simulink model "flow_sns"  (R2022a)
settings: Solver=FixedStepAuto  StartTime=0.0  StopTime=15  RelTol=1e-3  EnableMultiTasking=on
libraries: simulink x7, hdlsllib x4, mbedblockslib x3
settings Model: SimulationMode=external  ExtModeTrigDuration=10  Creator=FUGAZI  LastModifiedBy=smith
settings OptimizationCC: EnhancedBackFolding=on  PassReuseOutputArgsAs=Individual arguments  ZeroExternalMemoryAtStartup=off  ZeroInternalMemoryAtStartup=off  MaxStackSize=64  OptimizeBlockOrder=speed  DifferentSizesBufferReuse=on  OptimizationCustomize=off  EfficientTunableParamExpr=on
settings DebuggingCC: ParameterTunabilityLossMsg=error
settings HardwareCC: ProdBitPerPointer=32  ProdBitPerSizeT=32  ProdBitPerPtrDiffT=32  ProdLargestAtomicInteger=Long  ProdLargestAtomicFloat=Double  ProdWordSize=32  ProdLongLongMode=on  ProdHWDeviceType=ARM Compatible->ARM Cortex
settings SFSimCC: MATLABDynamicMemAlloc=off
settings RTWCC: SystemTargetFile=ert.tlc  HardwareBoard=STM32 Nucleo L476RG  TemplateMakefile=ert_default_tmf  Toolchain=GNU Tools for ARM Embedded Processors
settings CodeAppCC: ForceParamTrailComments=on  IgnoreCustomStorageClasses=off  OperatorAnnotations=on  SimulinkDataObjDesc=on  SFDataObjDesc=on  InsertBlockDesc=on
settings ERTTargetCC: SupportContinuousTime=on  ExtMode=on  ExtModeTransport=3  ExtModeStaticAlloc=on  ExtModeStaticAllocSize=2000  ExtModeMexFile=ext_xcp  ExtModeMexArgs=1 4 115200  ExtModeIntrfLevel=Level2 - Open

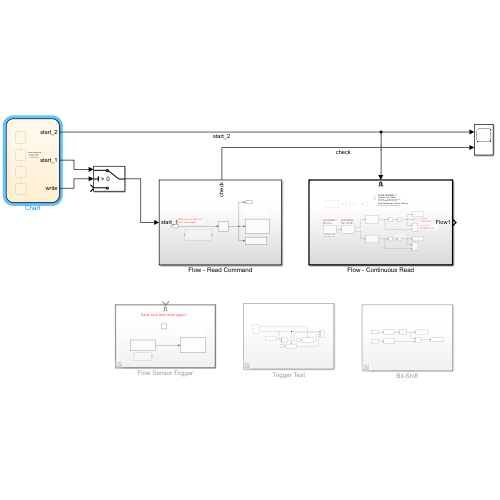
[thumbnail: Simulink's stored preview of the top-level diagram]
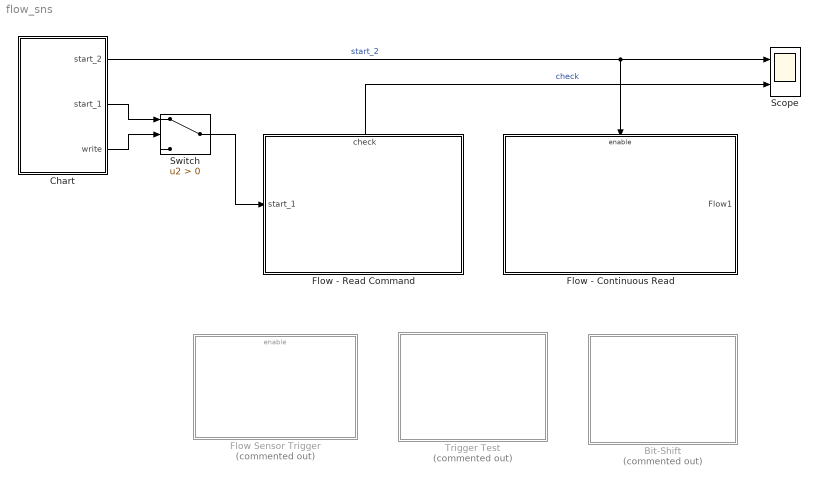
== system flow_sns ==
  Bit-Shift : Subsystem  Commented=on
  Chart : Stateflow chart  TreatAsAtomicUnit=on
      settings: PortSchema="{\"entries\":[{\"content\":{\"sides\":[{\"content\":{\"connectorIds\":[]},\"type\":\"ConnectorPlacement.EquallySpacedRectSide\",\"uuid\":\"751ec28f-069a-417f-8b9c-26d70f125eaf\"},{\"content\":{\"connectorIds\":[\"Out2\",\"Out1\",\"Out3\"],\"side\":\"RIGHT\"},\"type\":\"ConnectorPlacement.EquallySpacedRectSide\",\"uuid\":\"74ecb3a5-1f56-41c3-8a4c-212d8a69cc27\"},{\"content\":{\"connectorIds\":[],\"side\":\"TOP\"},\"type\":\"ConnectorPlacement.EquallySpacedRectSide\",\"uuid\":\"ea9723c7-ae57-446b-9b85-bce3bac5bf5f\"}]},\"type\":\"ConnectorPlacement.EquallySpacedConnector\",\"uuid\":\"1a0f9f5c-2546-4b71-a73d-7ce3ff689e76\"}],\"packageUris\":[\"http://schema.mathworks.com/mf0/Connector/R2020b\"],\"version\":\"1.0\"}"
  Flow - Continuous Read : Subsystem
  Flow - Read Command : Subsystem
      settings: PortSchema="{\"entries\":[{\"content\":{\"sides\":[{\"content\":{\"connectorIds\":[\"In1\"]},\"type\":\"ConnectorPlacement.EquallySpacedRectSide\",\"uuid\":\"93933be5-5d1d-4e29-9d84-8c5fcd33ad64\"},{\"content\":{\"connectorIds\":[],\"side\":\"RIGHT\"},\"type\":\"ConnectorPlacement.EquallySpacedRectSide\",\"uuid\":\"5f3334d1-31af-43f4-9ed8-c3b8fb739727\"},{\"content\":{\"connectorIds\":[\"Out1\"],\"side\":\"TOP\"},\"type\":\"ConnectorPlacement.EquallySpacedRectSide\",\"uuid\":\"aa0caa1c-490f-4eb3-a1f0-284b936a223e\"}]},\"type\":\"ConnectorPlacement.EquallySpacedConnector\",\"uuid\":\"c416ffdc-2385-461c-9877-3be2c663fd49\"}],\"packageUris\":[\"http://schema.mathworks.com/mf0/Connector/R2020b\"],\"version\":\"1.0\"}"
  Flow Sensor Trigger : Subsystem  Commented=on
  Scope : Scope  NumInputPorts=2
  Switch : Switch  Criteria=u2 > Threshold  SaturateOnIntegerOverflow=off  InputSameDT=off
  Trigger Test : Subsystem  Commented=on
  wires:
  Chart/1(start_1) -> Switch/1
  Chart/2(start_2) -> Flow - Continuous Read/Enable, Scope/1  "start_2"
  Switch/1 -> Flow - Read Command/1(start_1)
  Chart/3(write) -> Switch/2
  Flow - Read Command/1(check) -> Scope/2  "check"

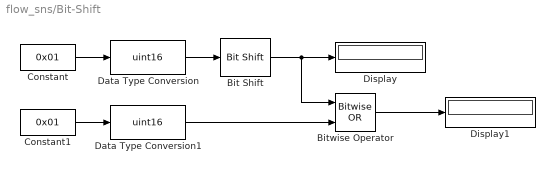
== system flow_sns/Bit-Shift ==
  Bit Shift : hdlsllib/Logic and Bit Operations/Bit Shift  mode=Shift Left Logical  N=8
  Bitwise Operator : simulink/Logic and Bit Operations/Bitwise Operator  logicop=OR  UseBitMask=off  NumInputPorts=2  BitMask=bin2dec('11011001')  BitMaskRealWorld=Stored Integer
  Constant : Constant  Value=0x01  SampleTime=0.1
  Constant1 : Constant  Value=0x01  SampleTime=0.1
  Data Type Conversion : DataTypeConversion  OutDataTypeStr=uint16  SaturateOnIntegerOverflow=off  RndMeth=Floor
  Data Type Conversion1 : DataTypeConversion  OutDataTypeStr=uint16  SaturateOnIntegerOverflow=off  RndMeth=Floor
  Display : Display
      settings: Format=hex (Stored Integer)
  Display1 : Display
      settings: Format=hex (Stored Integer)
  wires:
  Constant/1 -> Data Type Conversion/1
  Bit Shift/1 -> Bitwise Operator/1, Display/1
  Data Type Conversion/1 -> Bit Shift/1
  Constant1/1 -> Data Type Conversion1/1
  Bitwise Operator/1 -> Display1/1
  Data Type Conversion1/1 -> Bitwise Operator/2

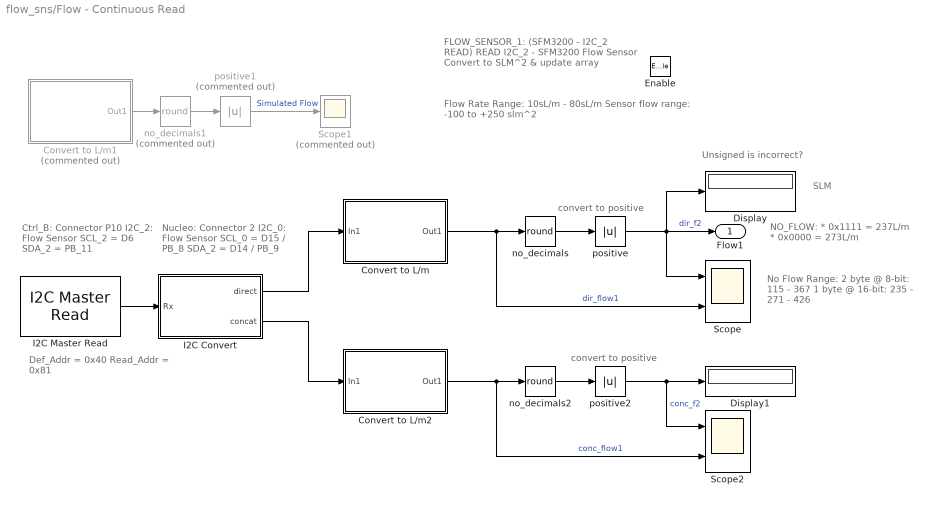
== system flow_sns/Flow - Continuous Read ==
  note: Unsigned is incorrect?
  note: NO_FLOW:
      | * 0x1111 = 237L/m
      | * 0x0000 = 273L/m
  note: Def_Addr = 0x40
      | Read_Addr = 0x81
  note: Ctrl_B: Connector P10
      | I2C_2: Flow Sensor
      | SCL_2 = D6
      | SDA_2 = PB_11
  note: FLOW_SENSOR_1:
      | (SFM3200 - I2C_2 READ)
      | READ I2C_2 - SFM3200 Flow Sensor
      | Convert to SLM^2 & update array
  note: SLM
  note: convert to positive
  note: Flow Rate Range: 10sL/m - 80sL/m
      | Sensor flow range: -100 to +250 slm^2
  note: Nucleo: Connector 2
      | I2C_0: Flow Sensor
      | SCL_0 = D15 / PB_8
      | SDA_2 = D14 / PB_9
  note: No Flow Range:
      | 2 byte @ 8-bit: 115 - 367
      | 1 byte @ 16-bit: 235 - 271 - 426
  note: convert to positive
  Enable : EnablePort
  Convert to L/m : Subsystem
  Convert to L/m1 : Subsystem  Commented=on
  Convert to L/m2 : Subsystem
  Display : Display
  Display1 : Display
  I2C Convert : Subsystem
  I2C Master Read : mbedblockslib/I2C Master Read  I2CModule=0  Mode=Master  SlaveAddress=hex2dec('81')  SlaveByteOrder=BigEndian  Direction=Receiver  RegisterAddressMode=off  RegisterAddress=uint8(0)  SlaveDataType=uint8  DataLength=3  NoAck=off  RepeatedStart=off  OutputStatus=off  SampleTime=0.1
      settings: SourceProductBaseCode=MICROBIT,NUCLEO,STMICRODIS
  Scope : Scope  NumInputPorts=2
  Scope1 : Scope  Commented=on
  Scope2 : Scope  NumInputPorts=2
  no_decimals : Rounding  Operator=round
  no_decimals1 : Rounding  Commented=on  Operator=round
  no_decimals2 : Rounding  Operator=round
  positive : Abs  SaturateOnIntegerOverflow=off
  positive1 : Abs  Commented=on  SaturateOnIntegerOverflow=off
  positive2 : Abs  SaturateOnIntegerOverflow=off
  Flow1 : Outport
  wires:
  no_decimals/1 -> positive/1
  positive/1 -> Display/1, Flow1/1, Scope/1  "dir_f2"
  I2C Master Read/1 -> I2C Convert/1(Rx)
  I2C Convert/1(direct) -> Convert to L/m/1(In1)
  Convert to L/m/1(Out1) -> Scope/2, no_decimals/1  "dir_flow1"
  no_decimals1/1 -> positive1/1
  Convert to L/m1/1(Out1) -> no_decimals1/1
  positive1/1 -> Scope1/1  "Simulated Flow"
  Convert to L/m2/1(Out1) -> Scope2/2, no_decimals2/1  "conc_flow1"
  I2C Convert/2(concat) -> Convert to L/m2/1(In1)
  no_decimals2/1 -> positive2/1
  positive2/1 -> Display1/1, Scope2/1  "conc_f2"

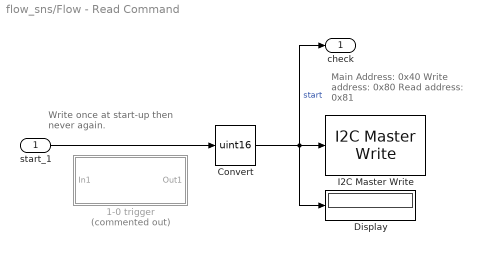
== system flow_sns/Flow - Read Command ==
  note: Main Address: 0x40
      | Write address: 0x80
      | Read address: 0x81
  note: Write once at start-up
      | then never again.
  start_1 : Inport
  1-0 trigger : Subsystem  Commented=on
  Convert : DataTypeConversion  OutDataTypeStr=uint16  RndMeth=Nearest  SaturateOnIntegerOverflow=off
  Display : Display
      settings: Format=hex (Stored Integer)
  I2C Master Write : mbedblockslib/I2C Master Write  I2CModule=0  Mode=Master  SlaveAddress=hex2dec('80')  SlaveByteOrder=BigEndian  Direction=Transmitter  RegisterAddressMode=off  RegisterAddress=uint8(1)  SlaveDataType=uint8  DataLength=2  NoAck=off  RepeatedStart=off  OutputStatus=off
      settings: SourceProductBaseCode=MICROBIT,NUCLEO,STMICRODIS
  check : Outport
  wires:
  start_1/1 -> Convert/1
  Convert/1 -> check/1, Display/1, I2C Master Write/1  "start"

== system flow_sns/Flow Sensor Trigger ==
  note: Send once then never again?
  note: Start continuous measurement
  note: Main Address: 0x40
      | Write address: 0x80
      | Read address: 0x81
  Enable : EnablePort
  Constant : Constant  Commented=on  Value=0x1000  SampleTime=-1
  Constant1 : Constant  Value=hex2dec('1000')  OutDataTypeStr=uint16
  I2C Master Write : mbedblockslib/I2C Master Write  I2CModule=0  Mode=Master  SlaveAddress=hex2dec('80')  SlaveByteOrder=BigEndian  Direction=Transmitter  RegisterAddressMode=off  RegisterAddress=uint8(1)  SlaveDataType=uint8  DataLength=2  NoAck=on  RepeatedStart=off  OutputStatus=off
      settings: SourceProductBaseCode=MICROBIT,NUCLEO,STMICRODIS
  wires:
  Constant1/1 -> I2C Master Write/1

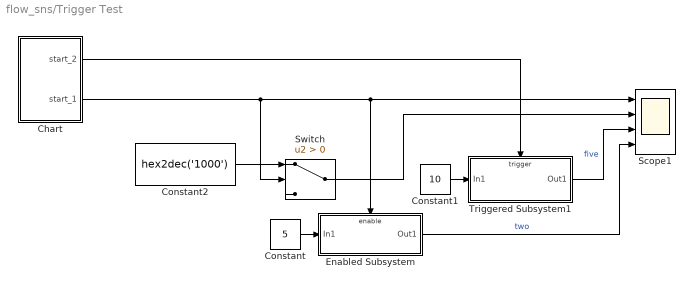
== system flow_sns/Trigger Test ==
  Chart : Stateflow chart  TreatAsAtomicUnit=on
      settings: PortSchema="{\"entries\":[{\"content\":{\"sides\":[{\"content\":{\"connectorIds\":[]},\"type\":\"ConnectorPlacement.EquallySpacedRectSide\",\"uuid\":\"751ec28f-069a-417f-8b9c-26d70f125eaf\"},{\"content\":{\"connectorIds\":[\"Out2\",\"Out1\"],\"side\":\"RIGHT\"},\"type\":\"ConnectorPlacement.EquallySpacedRectSide\",\"uuid\":\"74ecb3a5-1f56-41c3-8a4c-212d8a69cc27\"},{\"content\":{\"connectorIds\":[],\"side\":\"TOP\"},\"type\":\"ConnectorPlacement.EquallySpacedRectSide\",\"uuid\":\"ea9723c7-ae57-446b-9b85-bce3bac5bf5f\"}]},\"type\":\"ConnectorPlacement.EquallySpacedConnector\",\"uuid\":\"1a0f9f5c-2546-4b71-a73d-7ce3ff689e76\"}],\"packageUris\":[\"http://schema.mathworks.com/mf0/Connector/R2020b\"],\"version\":\"1.0\"}"
  Constant : Constant  Value=5
  Constant1 : Constant  Value=10
  Constant2 : Constant  Value=hex2dec('1000')  OutDataTypeStr=uint16
  Enabled Subsystem : Subsystem  TreatAsAtomicUnit=on
  Scope1 : Scope  NumInputPorts=4
  Switch : Switch  Criteria=u2 > Threshold  SaturateOnIntegerOverflow=off  InputSameDT=off
  Triggered Subsystem1 : Subsystem  TreatAsAtomicUnit=on
  wires:
  Constant/1 -> Enabled Subsystem/1(In1)
  Chart/2(start_2) -> Triggered Subsystem1/Trigger
  Constant1/1 -> Triggered Subsystem1/1(In1)
  Constant2/1 -> Switch/1
  Chart/1(start_1) -> Switch/2, Scope1/1, Enabled Subsystem/Enable
  Switch/1 -> Scope1/2
  Triggered Subsystem1/1(Out1) -> Scope1/3  "five"
  Enabled Subsystem/1(Out1) -> Scope1/4  "two"

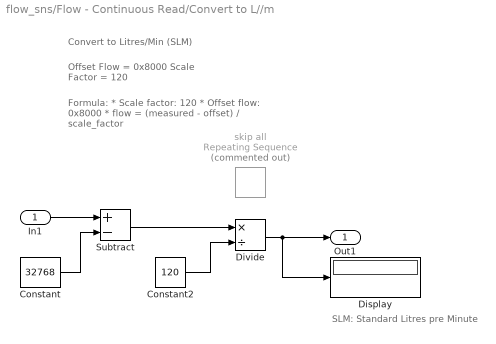
== system flow_sns/Flow - Continuous Read/Convert to L//m ==
  note: SLM: Standard Litres pre Minute
  note: Convert to Litres/Min (SLM)
  note: Offset Flow = 0x8000
      | Scale Factor = 120
  note: Formula:
      | * Scale factor: 120
      | * Offset flow: 0x8000
      | * flow = (measured - offset) / scale_factor
  In1 : Inport
  Constant : Constant  Value=32768
  Constant2 : Constant  Value=120
  Display : Display
  Divide : Product  Inputs=*/
  Subtract : Sum  Inputs=+-
  skip all : simulink/Sources/Repeating Sequence  Commented=on  rep_seq_t=[0 1.3 1.31 2.5 2.51]  rep_seq_y=[30 30 150 150 30]
  Out1 : Outport
  wires:
  Divide/1 -> Display/1, Out1/1
  Subtract/1 -> Divide/1
  Constant2/1 -> Divide/2
  Constant/1 -> Subtract/2
  In1/1 -> Subtract/1

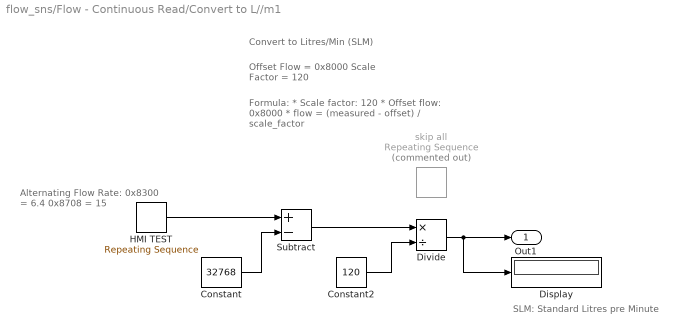
== system flow_sns/Flow - Continuous Read/Convert to L//m1 ==
  note: Formula:
      | * Scale factor: 120
      | * Offset flow: 0x8000
      | * flow = (measured - offset) / scale_factor
  note: Offset Flow = 0x8000
      | Scale Factor = 120
  note: Convert to Litres/Min (SLM)
  note: SLM: Standard Litres pre Minute
  note: Alternating Flow Rate:
      | 0x8300 = 6.4
      | 0x8708 = 15
  Constant : Constant  Value=32768
  Constant2 : Constant  Value=120
  Display : Display
  Divide : Product  Inputs=*/
  HMI TEST : simulink/Sources/Repeating Sequence  rep_seq_t=[0 2 2.05 4]  rep_seq_y=[0x8300 0x8300 0x8708 0x8708]
  Subtract : Sum  Inputs=+-
  skip all : simulink/Sources/Repeating Sequence  Commented=on  rep_seq_t=[0 1.3 1.31 2.5 2.51]  rep_seq_y=[30 30 150 150 30]
  Out1 : Outport
  wires:
  HMI TEST/1 -> Subtract/1
  Constant/1 -> Subtract/2
  Constant2/1 -> Divide/2
  Subtract/1 -> Divide/1
  Divide/1 -> Out1/1, Display/1

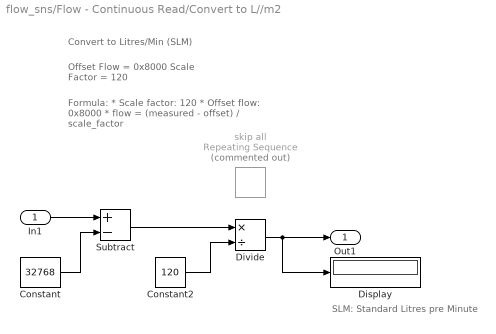
== system flow_sns/Flow - Continuous Read/Convert to L//m2 ==
  note: Formula:
      | * Scale factor: 120
      | * Offset flow: 0x8000
      | * flow = (measured - offset) / scale_factor
  note: Offset Flow = 0x8000
      | Scale Factor = 120
  note: Convert to Litres/Min (SLM)
  note: SLM: Standard Litres pre Minute
  In1 : Inport
  Constant : Constant  Value=32768
  Constant2 : Constant  Value=120
  Display : Display
  Divide : Product  Inputs=*/
  Subtract : Sum  Inputs=+-
  skip all : simulink/Sources/Repeating Sequence  Commented=on  rep_seq_t=[0 1.3 1.31 2.5 2.51]  rep_seq_y=[30 30 150 150 30]
  Out1 : Outport
  wires:
  In1/1 -> Subtract/1
  Constant/1 -> Subtract/2
  Constant2/1 -> Divide/2
  Subtract/1 -> Divide/1
  Divide/1 -> Out1/1, Display/1

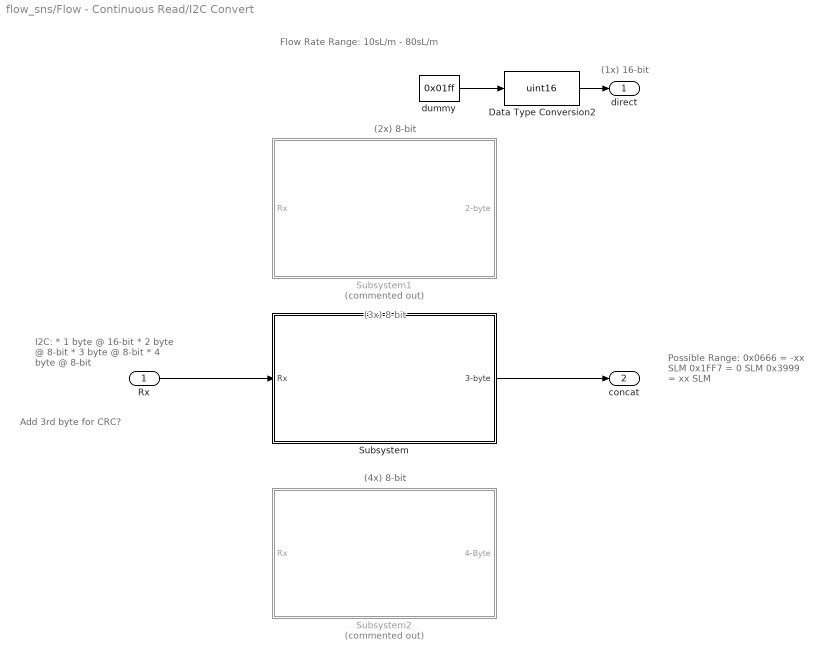
== system flow_sns/Flow - Continuous Read/I2C Convert ==
  note: (2x) 8-bit
  note: Possible Range:
      | 0x0666 = -xx SLM
      | 0x1FF7 = 0 SLM
      | 0x3999 = xx SLM
  note: Flow Rate Range: 10sL/m - 80sL/m
  note: I2C:
      | * 1 byte @ 16-bit
      | * 2 byte @ 8-bit
      | * 3 byte @ 8-bit
      | * 4 byte @ 8-bit
  note: (1x) 16-bit
  note: Add 3rd byte for CRC?
  note: (3x) 8-bit
  note: (4x) 8-bit
  Rx : Inport
  Data Type Conversion2 : DataTypeConversion  OutDataTypeStr=uint16  SaturateOnIntegerOverflow=off  RndMeth=Floor
  Subsystem : Subsystem
  Subsystem1 : Subsystem  Commented=on
  Subsystem2 : Subsystem  Commented=on
  dummy : Constant  Value=0x01ff
  direct : Outport
  concat : Outport  Port=2
  wires:
  Data Type Conversion2/1 -> direct/1
  dummy/1 -> Data Type Conversion2/1
  Rx/1 -> Subsystem/1(Rx)
  Subsystem/1(3-byte) -> concat/1

== system flow_sns/Flow - Read Command/1-0 trigger ==
  In1 : Inport
  Trigger Write : Switch  Criteria=u2 > Threshold  SaturateOnIntegerOverflow=off  InputSameDT=off
  dec(4096) : Constant  Value=hex2dec('1000')  OutDataTypeStr=uint16  SampleTime=0.1
  Out1 : Outport
  wires:
  dec(4096)/1 -> Trigger Write/1
  In1/1 -> Trigger Write/2
  Trigger Write/1 -> Out1/1

== system flow_sns/Trigger Test/Enabled Subsystem ==
  In1 : Inport
  Enable : EnablePort  StatesWhenEnabling=reset
  Out1 : Outport
  wires:
  In1/1 -> Out1/1

== system flow_sns/Trigger Test/Triggered Subsystem1 ==
  In1 : Inport
  Trigger : TriggerPort  VariantControl=(inherit)
  Constant : Constant  Value=5
  Out1 : Outport
  wires:
  In1/1 -> Out1/1

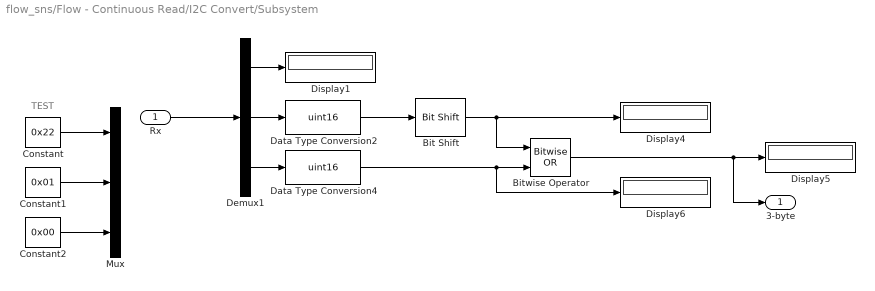
== system flow_sns/Flow - Continuous Read/I2C Convert/Subsystem ==
  note: TEST
  Rx : Inport
  Bit Shift : hdlsllib/Logic and Bit Operations/Bit Shift  mode=Shift Left Logical  N=8
  Bitwise Operator : simulink/Logic and Bit Operations/Bitwise Operator  logicop=OR  UseBitMask=off  NumInputPorts=2  BitMask=bin2dec('11011001')  BitMaskRealWorld=Stored Integer
  Constant : Constant  Value=0x22
  Constant1 : Constant  Value=0x01
  Constant2 : Constant  Value=0x00
  Data Type Conversion2 : DataTypeConversion  OutDataTypeStr=uint16  SaturateOnIntegerOverflow=off  RndMeth=Floor
  Data Type Conversion4 : DataTypeConversion  OutDataTypeStr=uint16  SaturateOnIntegerOverflow=off  RndMeth=Floor
  Demux1 : Demux  Outputs=3
  Display{1,4..6} (4 alike) : Display
      settings: Format=hex (Stored Integer)
  Mux : Mux  Inputs=3
  3-byte : Outport
  wires:
  Constant1/1 -> Mux/2
  Bit Shift/1 -> Bitwise Operator/1, Display4/1
  Demux1/3 -> Data Type Conversion4/1
  Data Type Conversion4/1 -> Display6/1, Bitwise Operator/2
  Bitwise Operator/1 -> 3-byte/1, Display5/1
  Data Type Conversion2/1 -> Bit Shift/1
  Demux1/2 -> Data Type Conversion2/1
  Demux1/1 -> Display1/1
  Constant2/1 -> Mux/3
  Constant/1 -> Mux/1
  Rx/1 -> Demux1/1

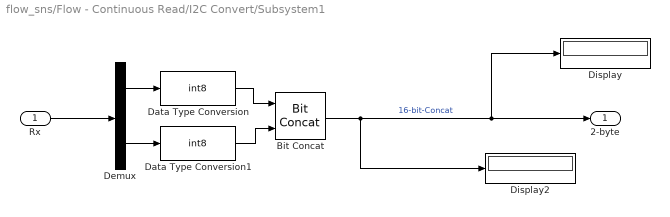
== system flow_sns/Flow - Continuous Read/I2C Convert/Subsystem1 ==
  Rx : Inport
  Bit Concat : hdlsllib/Logic and Bit Operations/Bit Concat  numInputs=2
  Data Type Conversion : DataTypeConversion  OutDataTypeStr=int8  SaturateOnIntegerOverflow=off  RndMeth=Floor
  Data Type Conversion1 : DataTypeConversion  OutDataTypeStr=int8  SaturateOnIntegerOverflow=off  RndMeth=Floor
  Demux : Demux  Outputs=2
  Display : Display
      settings: Format=hex (Stored Integer)
  Display2 : Display
      settings: Format=hex (Stored Integer)
  2-byte : Outport
  wires:
  Demux/2 -> Data Type Conversion1/1
  Bit Concat/1 -> 2-byte/1, Display/1, Display2/1  "16-bit-Concat"
  Data Type Conversion/1 -> Bit Concat/1
  Data Type Conversion1/1 -> Bit Concat/2
  Demux/1 -> Data Type Conversion/1
  Rx/1 -> Demux/1

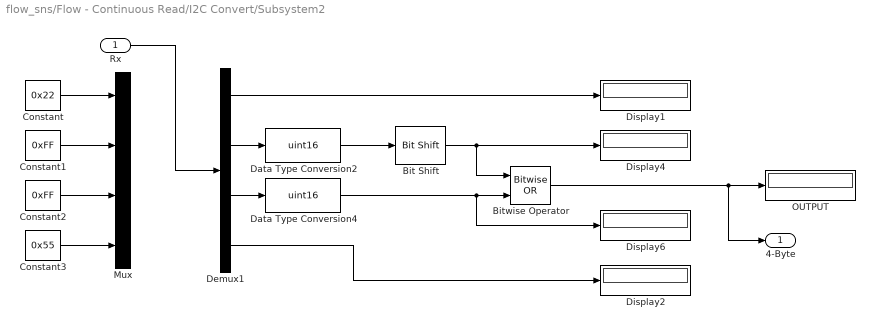
== system flow_sns/Flow - Continuous Read/I2C Convert/Subsystem2 ==
  Rx : Inport
  Bit Shift : hdlsllib/Logic and Bit Operations/Bit Shift  mode=Shift Left Logical  N=8
  Bitwise Operator : simulink/Logic and Bit Operations/Bitwise Operator  logicop=OR  UseBitMask=off  NumInputPorts=2  BitMask=bin2dec('11011001')  BitMaskRealWorld=Stored Integer
  Constant : Constant  Value=0x22
  Constant1 : Constant  Value=0xFF
  Constant2 : Constant  Value=0xFF
  Constant3 : Constant  Value=0x55
  Data Type Conversion2 : DataTypeConversion  OutDataTypeStr=uint16  SaturateOnIntegerOverflow=off  RndMeth=Floor
  Data Type Conversion4 : DataTypeConversion  OutDataTypeStr=uint16  SaturateOnIntegerOverflow=off  RndMeth=Floor
  Demux1 : Demux
  Display{1..2,4,6} (4 alike) : Display
      settings: Format=hex (Stored Integer)
  Mux : Mux
  OUTPUT : Display
      settings: Format=hex (Stored Integer)
  4-Byte : Outport
  wires:
  Constant/1 -> Mux/1
  Constant2/1 -> Mux/3
  Demux1/1 -> Display1/1
  Demux1/2 -> Data Type Conversion2/1
  Data Type Conversion2/1 -> Bit Shift/1
  Bitwise Operator/1 -> 4-Byte/1, OUTPUT/1
  Data Type Conversion4/1 -> Bitwise Operator/2, Display6/1
  Demux1/3 -> Data Type Conversion4/1
  Bit Shift/1 -> Display4/1, Bitwise Operator/1
  Constant1/1 -> Mux/2
  Constant3/1 -> Mux/4
  Demux1/4 -> Display2/1
  Rx/1 -> Demux1/1

== stateflow chart flow_sns/Chart ==
  state Initialise
    entry:
    start_1 = 0;
    start_2 = 0;
    write = 0;
    exit:
  state read1
    entry:
    write = 1;
    start_1 = 4096;
    start_2 = 0;
    exit:
  note: Read Commands:
      | * 0x31E3 - Offset
      | * 0x31E4 - Scale
      | * 0x1000 - READ
  state read2
    entry:
    write = 0;
    start_1 = 85;
    exit:
  state read3
    entry:
    start_2 = 1;
    exit:
  note: Start reading sensor after 100ms
  (default) -> Initialise
  Initialise -> read1 : after(50, msec)
  read1 -> read2 : after(25, msec)
  read2 -> read3 : after(75, msec)
  data: start_1 output; start_2 output; write output

== stateflow chart flow_sns/Trigger Test/Chart ==
  state Initialise
    entry:
    start_1 = 0;
    start_1 = 0;
    exit:
  state read
    entry:
    start_1 = 1;
    exit:
  state read1
    entry:
    start_1 = 0;
    start_2 = 1;
    exit:
  (default) -> Initialise
  Initialise -> read : after(100, msec)
  read -> read1 : after(100, msec)
  data: start_1 output; start_2 output
